simulink model "LoesungSimulink_MechanikR2020"  (R2020a)
settings: Solver=ode1  StartTime=0.0  StopTime=10.0  FixedStep=0.0001  RelTol=1e-3
undefined symbols (not defined in the file): D
settings Model: Creator=PM  LastModifiedBy=PM
settings DebuggingCC: UnconnectedInputMsg=none  UnconnectedOutputMsg=none  UnconnectedLineMsg=none
settings ModelReferenceCC: EnableRefExpFcnMdlSchedulingChecks=off
settings RTWCC: Description=Generic Real-Time Target

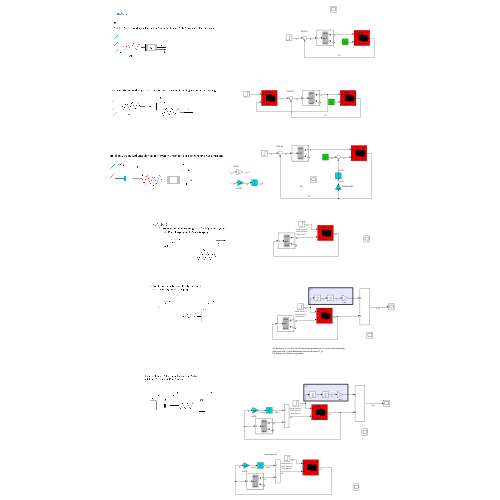
[thumbnail: Simulink's stored preview of the top-level diagram]
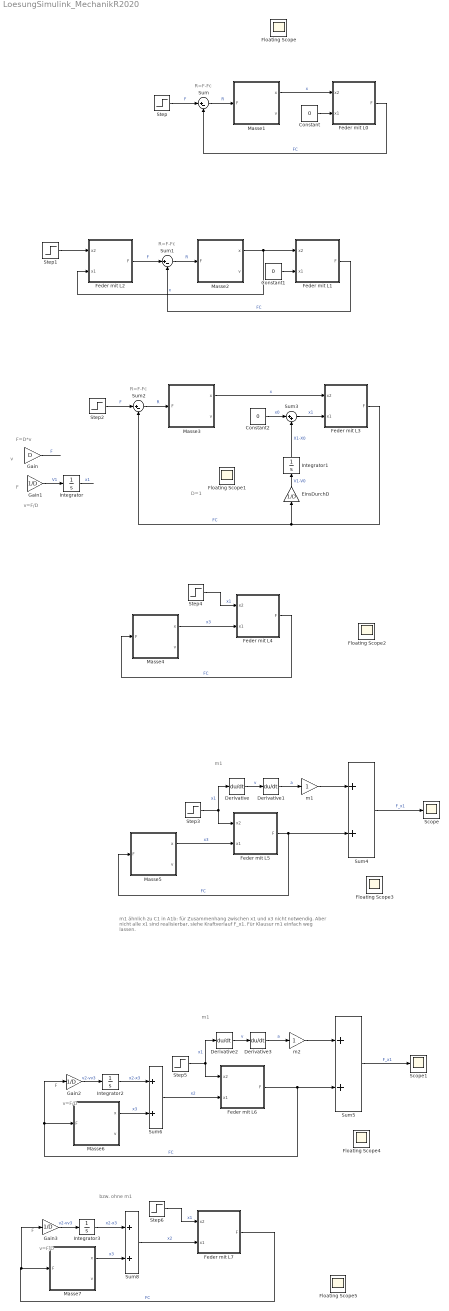
== system LoesungSimulink_MechanikR2020 ==
  note: m1
  note: m1 ähnlich zu C1 in  A1b: für Zusammenhang zwischen x1 und x3 nicht notwendig.
      | Aber nicht alle x1 sind realisierbar, siehe Kraftverlauf F_x1.
      | Für Klausur m1 einfach weg lassen.
  note: D=1
  note: F=D*v
  note: F
  note: v
  note: R=F-Fc
  note: R=F-Fc
  note: R=F-Fc
  note: v=F/D
  note: m1
  note: bzw. ohne m1
  note: F
  note: v=F/D
  note: F
  note: v=F/D
  " Feder mit L0" : Subsystem  mask{C=1, L0=0}
      mask prompts: C "Spring Constant C [N/m]"; L0 "Length of Spring if no force is applied L0 [m]"
      mask help:
      | If no force F is applied, the spring has the length L0.
      |
      | F=C*sign(x2-x1-L0)*((x2-x1-L0)
      mask Display:
      | plot(20,0)
      | plot(90,100)
      | plot([60,60],[25,30])
      | plot([60,80],[30,32])
      | plot([80,40],[32,36])
      | plot([40,80],[36,40])
      | plot([80,40],[40,44])
      | plot([40,80],[44,48])
      | plot([80,40],[48,52])
      | plot([40,80],[52,56])
      | plot([80,40],[56,60])
      | plot([40,80],[60,64])
      | plot([80,40],[64,68])
      | plot([40,60],[68,70])
      | plot([60,60],[70,75])
      | 
      | 
      | port_label ('output',1,'F')
      | port_label ('input',1,'x2')
      | port_label ('input',2,'x1')
      | 
      | text(40,10,['C=',num2str(C)])
      | text(40,90,['L0=',num2str(L0)])
  " Feder mit L1" : Subsystem  mask{C=1, L0=0}
      mask prompts: C "Spring Constant C [N/m]"; L0 "Length of Spring if no force is applied L0 [m]"
      mask help:
      | If no force F is applied, the spring has the length L0.
      |
      | F=C*sign(x2-x1-L0)*((x2-x1-L0)
      mask Display:
      | plot(20,0)
      | plot(90,100)
      | plot([60,60],[25,30])
      | plot([60,80],[30,32])
      | plot([80,40],[32,36])
      | plot([40,80],[36,40])
      | plot([80,40],[40,44])
      | plot([40,80],[44,48])
      | plot([80,40],[48,52])
      | plot([40,80],[52,56])
      | plot([80,40],[56,60])
      | plot([40,80],[60,64])
      | plot([80,40],[64,68])
      | plot([40,60],[68,70])
      | plot([60,60],[70,75])
      | 
      | 
      | port_label ('output',1,'F')
      | port_label ('input',1,'x2')
      | port_label ('input',2,'x1')
      | 
      | text(40,10,['C=',num2str(C)])
      | text(40,90,['L0=',num2str(L0)])
  " Feder mit L2" : Subsystem  mask{C=1, L0=0}
      mask prompts: C "Spring Constant C [N/m]"; L0 "Length of Spring if no force is applied L0 [m]"
      mask help:
      | If no force F is applied, the spring has the length L0.
      |
      | F=C*sign(x2-x1-L0)*((x2-x1-L0)
      mask Display:
      | plot(20,0)
      | plot(90,100)
      | plot([60,60],[25,30])
      | plot([60,80],[30,32])
      | plot([80,40],[32,36])
      | plot([40,80],[36,40])
      | plot([80,40],[40,44])
      | plot([40,80],[44,48])
      | plot([80,40],[48,52])
      | plot([40,80],[52,56])
      | plot([80,40],[56,60])
      | plot([40,80],[60,64])
      | plot([80,40],[64,68])
      | plot([40,60],[68,70])
      | plot([60,60],[70,75])
      | 
      | 
      | port_label ('output',1,'F')
      | port_label ('input',1,'x2')
      | port_label ('input',2,'x1')
      | 
      | text(40,10,['C=',num2str(C)])
      | text(40,90,['L0=',num2str(L0)])
  " Feder mit L3" : Subsystem  mask{C=1, L0=0}
      mask prompts: C "Spring Constant C [N/m]"; L0 "Length of Spring if no force is applied L0 [m]"
      mask help:
      | If no force F is applied, the spring has the length L0.
      |
      | F=C*sign(x2-x1-L0)*((x2-x1-L0)
      mask Display:
      | plot(20,0)
      | plot(90,100)
      | plot([60,60],[25,30])
      | plot([60,80],[30,32])
      | plot([80,40],[32,36])
      | plot([40,80],[36,40])
      | plot([80,40],[40,44])
      | plot([40,80],[44,48])
      | plot([80,40],[48,52])
      | plot([40,80],[52,56])
      | plot([80,40],[56,60])
      | plot([40,80],[60,64])
      | plot([80,40],[64,68])
      | plot([40,60],[68,70])
      | plot([60,60],[70,75])
      | 
      | 
      | port_label ('output',1,'F')
      | port_label ('input',1,'x2')
      | port_label ('input',2,'x1')
      | 
      | text(40,10,['C=',num2str(C)])
      | text(40,90,['L0=',num2str(L0)])
  " Feder mit L4" : Subsystem  mask{C=1, L0=1}
      mask prompts: C "Spring Constant C [N/m]"; L0 "Length of Spring if no force is applied L0 [m]"
      mask help:
      | If no force F is applied, the spring has the length L0.
      |
      | F=C*sign(x2-x1-L0)*((x2-x1-L0)
      mask Display:
      | plot(20,0)
      | plot(90,100)
      | plot([60,60],[25,30])
      | plot([60,80],[30,32])
      | plot([80,40],[32,36])
      | plot([40,80],[36,40])
      | plot([80,40],[40,44])
      | plot([40,80],[44,48])
      | plot([80,40],[48,52])
      | plot([40,80],[52,56])
      | plot([80,40],[56,60])
      | plot([40,80],[60,64])
      | plot([80,40],[64,68])
      | plot([40,60],[68,70])
      | plot([60,60],[70,75])
      | 
      | 
      | port_label ('output',1,'F')
      | port_label ('input',1,'x2')
      | port_label ('input',2,'x1')
      | 
      | text(40,10,['C=',num2str(C)])
      | text(40,90,['L0=',num2str(L0)])
  " Feder mit L5" : Subsystem  mask{C=1, L0=1}
      mask prompts: C "Spring Constant C [N/m]"; L0 "Length of Spring if no force is applied L0 [m]"
      mask help:
      | If no force F is applied, the spring has the length L0.
      |
      | F=C*sign(x2-x1-L0)*((x2-x1-L0)
      mask Display:
      | plot(20,0)
      | plot(90,100)
      | plot([60,60],[25,30])
      | plot([60,80],[30,32])
      | plot([80,40],[32,36])
      | plot([40,80],[36,40])
      | plot([80,40],[40,44])
      | plot([40,80],[44,48])
      | plot([80,40],[48,52])
      | plot([40,80],[52,56])
      | plot([80,40],[56,60])
      | plot([40,80],[60,64])
      | plot([80,40],[64,68])
      | plot([40,60],[68,70])
      | plot([60,60],[70,75])
      | 
      | 
      | port_label ('output',1,'F')
      | port_label ('input',1,'x2')
      | port_label ('input',2,'x1')
      | 
      | text(40,10,['C=',num2str(C)])
      | text(40,90,['L0=',num2str(L0)])
  " Feder mit L6" : Subsystem  mask{C=1, L0=1}
      mask prompts: C "Spring Constant C [N/m]"; L0 "Length of Spring if no force is applied L0 [m]"
      mask help:
      | If no force F is applied, the spring has the length L0.
      |
      | F=C*sign(x2-x1-L0)*((x2-x1-L0)
      mask Display:
      | plot(20,0)
      | plot(90,100)
      | plot([60,60],[25,30])
      | plot([60,80],[30,32])
      | plot([80,40],[32,36])
      | plot([40,80],[36,40])
      | plot([80,40],[40,44])
      | plot([40,80],[44,48])
      | plot([80,40],[48,52])
      | plot([40,80],[52,56])
      | plot([80,40],[56,60])
      | plot([40,80],[60,64])
      | plot([80,40],[64,68])
      | plot([40,60],[68,70])
      | plot([60,60],[70,75])
      | 
      | 
      | port_label ('output',1,'F')
      | port_label ('input',1,'x2')
      | port_label ('input',2,'x1')
      | 
      | text(40,10,['C=',num2str(C)])
      | text(40,90,['L0=',num2str(L0)])
  " Feder mit L7" : Subsystem  mask{C=1, L0=1}
      mask prompts: C "Spring Constant C [N/m]"; L0 "Length of Spring if no force is applied L0 [m]"
      mask help:
      | If no force F is applied, the spring has the length L0.
      |
      | F=C*sign(x2-x1-L0)*((x2-x1-L0)
      mask Display:
      | plot(20,0)
      | plot(90,100)
      | plot([60,60],[25,30])
      | plot([60,80],[30,32])
      | plot([80,40],[32,36])
      | plot([40,80],[36,40])
      | plot([80,40],[40,44])
      | plot([40,80],[44,48])
      | plot([80,40],[48,52])
      | plot([40,80],[52,56])
      | plot([80,40],[56,60])
      | plot([40,80],[60,64])
      | plot([80,40],[64,68])
      | plot([40,60],[68,70])
      | plot([60,60],[70,75])
      | 
      | 
      | port_label ('output',1,'F')
      | port_label ('input',1,'x2')
      | port_label ('input',2,'x1')
      | 
      | text(40,10,['C=',num2str(C)])
      | text(40,90,['L0=',num2str(L0)])
  Constant : Constant  Value=0
  Constant1 : Constant  Value=0
  Constant2 : Constant  Value=0
  Derivative{,1..3} (4 alike) : Derivative
  EinsDurchD : Gain  Gain=1/D
  Floating Scope{,1..5} (6 alike) : Scope
      settings: Floating=on
  Gain : Gain  Gain=D
  Gain1 : Gain  Gain=1/D
  Gain2 : Gain  Gain=1/D
  Gain3 : Gain  Gain=1/D
  Integrator{,1..3} (4 alike) : Integrator
  Masse1 : Subsystem  mask{m=1, v0=0, x0=0}
      mask prompts: m "Masse m"; v0 "Anfangsgeschwindigkeit v_0"; x0 "Anfangsposition x_0"
      mask help:
      | Calculates the position s and the velocity v of a mass as a function of the Force F and the initial velocity v_0 and initial position s_0.
      | Berechnet die Position und die Geschwindigkeit eines Köpers mit der Masse m. Auf den Köper wirkt die Kraft F. Die Anfangsposition ist s_0, die Anfangsgeschwindigkeit ist v_0.
      mask Display:
      | plot(0,0)
      | plot(100,100)
      | patch([35 35 70 70],[10 90 90 10],[0.7,0.7,0.7])
      | text(40,80,['x0=',num2str(x0)])
      | text(40,50,['m=',num2str(m)])
      | text(40,20,['v0=',num2str(v0)])
      | plot([70 80],[70 70])
      | patch([80 80 85],[65 75 70],[0 0 0])
      | plot([15 35],[50 50])
      | patch([30 30 35],[45 55 50],[0 0 0])
      | plot([70 80],[30 30])
      | patch([80 80 85],[25 35 30],[0 0 0])
      | port_label ('output',1,'x')
      | port_label ('output',2,'v')
      | port_label ('input',1,'F')
  Masse2 : Subsystem  mask{m=1, v0=0, x0=0}
      mask prompts: m "Masse m"; v0 "Anfangsgeschwindigkeit v_0"; x0 "Anfangsposition x_0"
      mask help:
      | Calculates the position s and the velocity v of a mass as a function of the Force F and the initial velocity v_0 and initial position s_0.
      | Berechnet die Position und die Geschwindigkeit eines Köpers mit der Masse m. Auf den Köper wirkt die Kraft F. Die Anfangsposition ist s_0, die Anfangsgeschwindigkeit ist v_0.
      mask Display:
      | plot(0,0)
      | plot(100,100)
      | patch([35 35 70 70],[10 90 90 10],[0.7,0.7,0.7])
      | text(40,80,['x0=',num2str(x0)])
      | text(40,50,['m=',num2str(m)])
      | text(40,20,['v0=',num2str(v0)])
      | plot([70 80],[70 70])
      | patch([80 80 85],[65 75 70],[0 0 0])
      | plot([15 35],[50 50])
      | patch([30 30 35],[45 55 50],[0 0 0])
      | plot([70 80],[30 30])
      | patch([80 80 85],[25 35 30],[0 0 0])
      | port_label ('output',1,'x')
      | port_label ('output',2,'v')
      | port_label ('input',1,'F')
  Masse3 : Subsystem  mask{m=1, v0=0, x0=0}
      mask prompts: m "Masse m"; v0 "Anfangsgeschwindigkeit v_0"; x0 "Anfangsposition x_0"
      mask help:
      | Calculates the position s and the velocity v of a mass as a function of the Force F and the initial velocity v_0 and initial position s_0.
      | Berechnet die Position und die Geschwindigkeit eines Köpers mit der Masse m. Auf den Köper wirkt die Kraft F. Die Anfangsposition ist s_0, die Anfangsgeschwindigkeit ist v_0.
      mask Display:
      | plot(0,0)
      | plot(100,100)
      | patch([35 35 70 70],[10 90 90 10],[0.7,0.7,0.7])
      | text(40,80,['x0=',num2str(x0)])
      | text(40,50,['m=',num2str(m)])
      | text(40,20,['v0=',num2str(v0)])
      | plot([70 80],[70 70])
      | patch([80 80 85],[65 75 70],[0 0 0])
      | plot([15 35],[50 50])
      | patch([30 30 35],[45 55 50],[0 0 0])
      | plot([70 80],[30 30])
      | patch([80 80 85],[25 35 30],[0 0 0])
      | port_label ('output',1,'x')
      | port_label ('output',2,'v')
      | port_label ('input',1,'F')
  Masse4 : Subsystem  mask{m=1, v0=0, x0=0}
      mask prompts: m "Masse m"; v0 "Anfangsgeschwindigkeit v_0"; x0 "Anfangsposition x_0"
      mask help:
      | Calculates the position s and the velocity v of a mass as a function of the Force F and the initial velocity v_0 and initial position s_0.
      | Berechnet die Position und die Geschwindigkeit eines Köpers mit der Masse m. Auf den Köper wirkt die Kraft F. Die Anfangsposition ist s_0, die Anfangsgeschwindigkeit ist v_0.
      mask Display:
      | plot(0,0)
      | plot(100,100)
      | patch([35 35 70 70],[10 90 90 10],[0.7,0.7,0.7])
      | text(40,80,['x0=',num2str(x0)])
      | text(40,50,['m=',num2str(m)])
      | text(40,20,['v0=',num2str(v0)])
      | plot([70 80],[70 70])
      | patch([80 80 85],[65 75 70],[0 0 0])
      | plot([15 35],[50 50])
      | patch([30 30 35],[45 55 50],[0 0 0])
      | plot([70 80],[30 30])
      | patch([80 80 85],[25 35 30],[0 0 0])
      | port_label ('output',1,'x')
      | port_label ('output',2,'v')
      | port_label ('input',1,'F')
  Masse5 : Subsystem  mask{m=1, v0=0, x0=0}
      mask prompts: m "Masse m"; v0 "Anfangsgeschwindigkeit v_0"; x0 "Anfangsposition x_0"
      mask help:
      | Calculates the position s and the velocity v of a mass as a function of the Force F and the initial velocity v_0 and initial position s_0.
      | Berechnet die Position und die Geschwindigkeit eines Köpers mit der Masse m. Auf den Köper wirkt die Kraft F. Die Anfangsposition ist s_0, die Anfangsgeschwindigkeit ist v_0.
      mask Display:
      | plot(0,0)
      | plot(100,100)
      | patch([35 35 70 70],[10 90 90 10],[0.7,0.7,0.7])
      | text(40,80,['x0=',num2str(x0)])
      | text(40,50,['m=',num2str(m)])
      | text(40,20,['v0=',num2str(v0)])
      | plot([70 80],[70 70])
      | patch([80 80 85],[65 75 70],[0 0 0])
      | plot([15 35],[50 50])
      | patch([30 30 35],[45 55 50],[0 0 0])
      | plot([70 80],[30 30])
      | patch([80 80 85],[25 35 30],[0 0 0])
      | port_label ('output',1,'x')
      | port_label ('output',2,'v')
      | port_label ('input',1,'F')
  Masse6 : Subsystem  mask{m=1, v0=0, x0=0}
      mask prompts: m "Masse m"; v0 "Anfangsgeschwindigkeit v_0"; x0 "Anfangsposition x_0"
      mask help:
      | Calculates the position s and the velocity v of a mass as a function of the Force F and the initial velocity v_0 and initial position s_0.
      | Berechnet die Position und die Geschwindigkeit eines Köpers mit der Masse m. Auf den Köper wirkt die Kraft F. Die Anfangsposition ist s_0, die Anfangsgeschwindigkeit ist v_0.
      mask Display:
      | plot(0,0)
      | plot(100,100)
      | patch([35 35 70 70],[10 90 90 10],[0.7,0.7,0.7])
      | text(40,80,['x0=',num2str(x0)])
      | text(40,50,['m=',num2str(m)])
      | text(40,20,['v0=',num2str(v0)])
      | plot([70 80],[70 70])
      | patch([80 80 85],[65 75 70],[0 0 0])
      | plot([15 35],[50 50])
      | patch([30 30 35],[45 55 50],[0 0 0])
      | plot([70 80],[30 30])
      | patch([80 80 85],[25 35 30],[0 0 0])
      | port_label ('output',1,'x')
      | port_label ('output',2,'v')
      | port_label ('input',1,'F')
  Masse7 : Subsystem  mask{m=1, v0=0, x0=0}
      mask prompts: m "Masse m"; v0 "Anfangsgeschwindigkeit v_0"; x0 "Anfangsposition x_0"
      mask help:
      | Calculates the position s and the velocity v of a mass as a function of the Force F and the initial velocity v_0 and initial position s_0.
      | Berechnet die Position und die Geschwindigkeit eines Köpers mit der Masse m. Auf den Köper wirkt die Kraft F. Die Anfangsposition ist s_0, die Anfangsgeschwindigkeit ist v_0.
      mask Display:
      | plot(0,0)
      | plot(100,100)
      | patch([35 35 70 70],[10 90 90 10],[0.7,0.7,0.7])
      | text(40,80,['x0=',num2str(x0)])
      | text(40,50,['m=',num2str(m)])
      | text(40,20,['v0=',num2str(v0)])
      | plot([70 80],[70 70])
      | patch([80 80 85],[65 75 70],[0 0 0])
      | plot([15 35],[50 50])
      | patch([30 30 35],[45 55 50],[0 0 0])
      | plot([70 80],[30 30])
      | patch([80 80 85],[25 35 30],[0 0 0])
      | port_label ('output',1,'x')
      | port_label ('output',2,'v')
      | port_label ('input',1,'F')
  Scope : Scope
  Scope1 : Scope
  Step : Step  SampleTime=0
  Step1 : Step  SampleTime=0
  Step2 : Step  SampleTime=0
  Step{3..6} (4 alike) : Step  Before=1  After=2  SampleTime=0
      settings: AttributesFormatString=initial value=%<Before>\nfinal value=%<After>\nstep time=%<Time>
  Sum : Sum  Inputs=|+-
  Sum1 : Sum  Inputs=|+-
  Sum2 : Sum  Inputs=|+-
  Sum3 : Sum  Inputs=|++
  Sum{4..6,8} (4 alike) : Sum
  m1 : Gain
  m2 : Gain
  wires:
  Constant/1 -> " Feder mit L0"/2(x1)
  Masse1/1(x) -> " Feder mit L0"/1(x2)  "x"
  Sum/1 -> Masse1/1(F)  "R"
  Step/1 -> Sum/1  "F"
  " Feder mit L0"/1(F) -> Sum/2  "FC"
  Constant1/1 -> " Feder mit L1"/2(x1)
  " Feder mit L1"/1(F) -> Sum1/2  "FC"
  Sum1/1 -> Masse2/1(F)  "R"
  Masse2/1(x) -> " Feder mit L2"/2(x1), " Feder mit L1"/1(x2)  "x"
  " Feder mit L2"/1(F) -> Sum1/1  "F"
  Step1/1 -> " Feder mit L2"/1(x2)
  " Feder mit L3"/1(F) -> EinsDurchD/1, Sum2/2  "FC"
  Sum2/1 -> Masse3/1(F)  "R"
  Masse3/1(x) -> " Feder mit L3"/1(x2)  "x"
  Step2/1 -> Sum2/1  "F"
  ? -> Gain/1
  Gain/1 -> ?  "F"
  ? -> Gain1/1
  Gain1/1 -> Integrator/1  "V1"
  Integrator/1 -> ?  "x1"
  EinsDurchD/1 -> Integrator1/1  "V1-V0"
  Sum3/1 -> " Feder mit L3"/2(x1)  "x1"
  Integrator1/1 -> Sum3/2  "X1-X0"
  Constant2/1 -> Sum3/1  "x0"
  Masse4/1(x) -> " Feder mit L4"/2(x1)  "x3"
  Step4/1 -> " Feder mit L4"/1(x2)  "x1"
  " Feder mit L4"/1(F) -> Masse4/1(F)  "FC"
  Step3/1 -> " Feder mit L5"/1(x2), Derivative/1  "x1"
  Masse5/1(x) -> " Feder mit L5"/2(x1)  "x3"
  " Feder mit L5"/1(F) -> Sum4/2, Masse5/1(F)  "FC"
  Derivative/1 -> Derivative1/1  "v"
  Derivative1/1 -> m1/1  "a"
  m1/1 -> Sum4/1
  Sum4/1 -> Scope/1  "F_x1"
  Sum5/1 -> Scope1/1  "F_x1"
  m2/1 -> Sum5/1
  Derivative3/1 -> m2/1  "a"
  " Feder mit L6"/1(F) -> Gain2/1, Masse6/1(F), Sum5/2  "FC"
  Sum6/1 -> " Feder mit L6"/2(x1)  "x2"
  Step5/1 -> " Feder mit L6"/1(x2), Derivative2/1  "x1"
  Derivative2/1 -> Derivative3/1  "v"
  Integrator2/1 -> Sum6/1  "x2-x3"
  Gain2/1 -> Integrator2/1  "v2-vv3"
  Masse6/1(x) -> Sum6/2  "x3"
  Integrator3/1 -> Sum8/1  "x2-x3"
  Gain3/1 -> Integrator3/1  "v2-vv3"
  " Feder mit L7"/1(F) -> Gain3/1, Masse7/1(F)  "FC"
  Masse7/1(x) -> Sum8/2  "x3"
  Step6/1 -> " Feder mit L7"/1(x2)  "x1"
  Sum8/1 -> " Feder mit L7"/2(x1)  "x2"

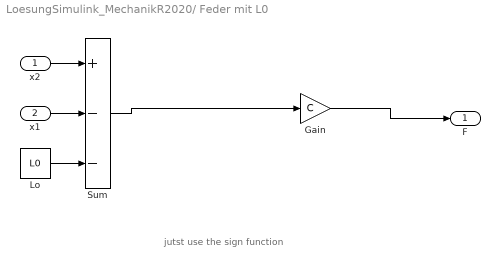
== system LoesungSimulink_MechanikR2020/ Feder mit L0 ==
  note: jutst use the sign function
  x2 : Inport
  x1 : Inport  Port=2
  Gain : Gain  Gain=C
  Lo : Constant  Value=L0
  Sum : Sum  Inputs=+--
  F : Outport  VectorParamsAs1DForOutWhenUnconnected=off
  wires:
  Gain/1 -> F/1
  Sum/1 -> Gain/1
  Lo/1 -> Sum/3
  x1/1 -> Sum/2
  x2/1 -> Sum/1

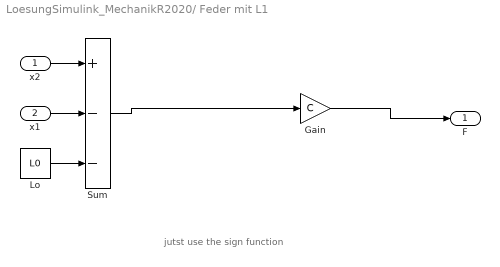
== system LoesungSimulink_MechanikR2020/ Feder mit L1 ==
  note: jutst use the sign function
  x2 : Inport
  x1 : Inport  Port=2
  Gain : Gain  Gain=C
  Lo : Constant  Value=L0
  Sum : Sum  Inputs=+--
  F : Outport  VectorParamsAs1DForOutWhenUnconnected=off
  wires:
  Gain/1 -> F/1
  Sum/1 -> Gain/1
  Lo/1 -> Sum/3
  x1/1 -> Sum/2
  x2/1 -> Sum/1

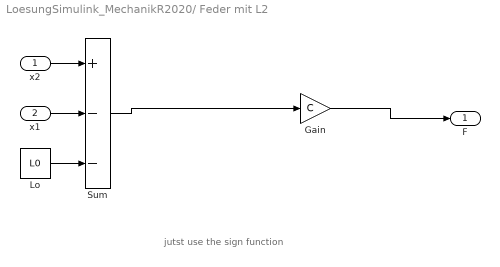
== system LoesungSimulink_MechanikR2020/ Feder mit L2 ==
  note: jutst use the sign function
  x2 : Inport
  x1 : Inport  Port=2
  Gain : Gain  Gain=C
  Lo : Constant  Value=L0
  Sum : Sum  Inputs=+--
  F : Outport  VectorParamsAs1DForOutWhenUnconnected=off
  wires:
  Gain/1 -> F/1
  Sum/1 -> Gain/1
  Lo/1 -> Sum/3
  x1/1 -> Sum/2
  x2/1 -> Sum/1

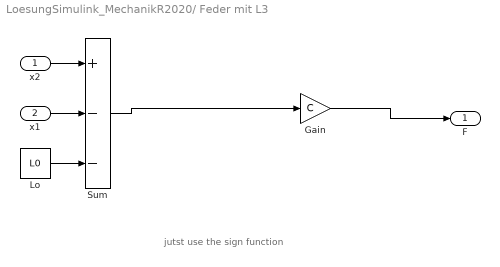
== system LoesungSimulink_MechanikR2020/ Feder mit L3 ==
  note: jutst use the sign function
  x2 : Inport
  x1 : Inport  Port=2
  Gain : Gain  Gain=C
  Lo : Constant  Value=L0
  Sum : Sum  Inputs=+--
  F : Outport  VectorParamsAs1DForOutWhenUnconnected=off
  wires:
  Gain/1 -> F/1
  Sum/1 -> Gain/1
  Lo/1 -> Sum/3
  x1/1 -> Sum/2
  x2/1 -> Sum/1

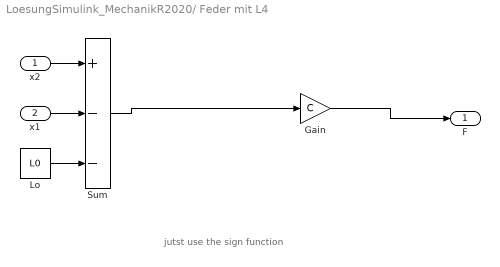
== system LoesungSimulink_MechanikR2020/ Feder mit L4 ==
  note: jutst use the sign function
  x2 : Inport
  x1 : Inport  Port=2
  Gain : Gain  Gain=C
  Lo : Constant  Value=L0
  Sum : Sum  Inputs=+--
  F : Outport  VectorParamsAs1DForOutWhenUnconnected=off
  wires:
  Gain/1 -> F/1
  Sum/1 -> Gain/1
  Lo/1 -> Sum/3
  x1/1 -> Sum/2
  x2/1 -> Sum/1

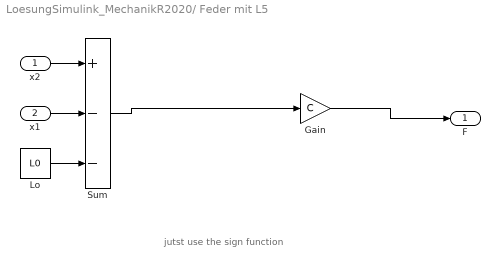
== system LoesungSimulink_MechanikR2020/ Feder mit L5 ==
  note: jutst use the sign function
  x2 : Inport
  x1 : Inport  Port=2
  Gain : Gain  Gain=C
  Lo : Constant  Value=L0
  Sum : Sum  Inputs=+--
  F : Outport  VectorParamsAs1DForOutWhenUnconnected=off
  wires:
  Gain/1 -> F/1
  Sum/1 -> Gain/1
  Lo/1 -> Sum/3
  x1/1 -> Sum/2
  x2/1 -> Sum/1

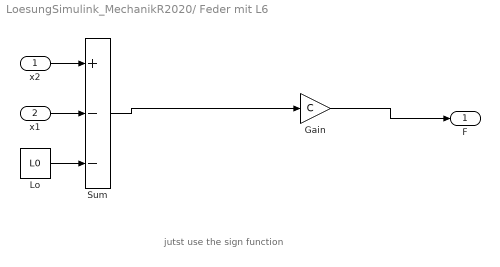
== system LoesungSimulink_MechanikR2020/ Feder mit L6 ==
  note: jutst use the sign function
  x2 : Inport
  x1 : Inport  Port=2
  Gain : Gain  Gain=C
  Lo : Constant  Value=L0
  Sum : Sum  Inputs=+--
  F : Outport  VectorParamsAs1DForOutWhenUnconnected=off
  wires:
  Gain/1 -> F/1
  Sum/1 -> Gain/1
  Lo/1 -> Sum/3
  x1/1 -> Sum/2
  x2/1 -> Sum/1

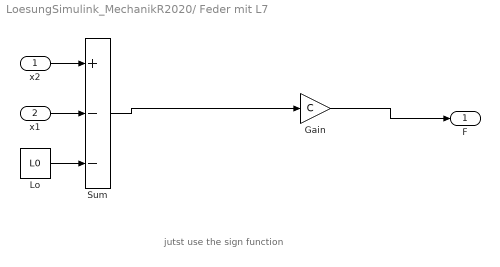
== system LoesungSimulink_MechanikR2020/ Feder mit L7 ==
  note: jutst use the sign function
  x2 : Inport
  x1 : Inport  Port=2
  Gain : Gain  Gain=C
  Lo : Constant  Value=L0
  Sum : Sum  Inputs=+--
  F : Outport  VectorParamsAs1DForOutWhenUnconnected=off
  wires:
  Gain/1 -> F/1
  Sum/1 -> Gain/1
  Lo/1 -> Sum/3
  x1/1 -> Sum/2
  x2/1 -> Sum/1

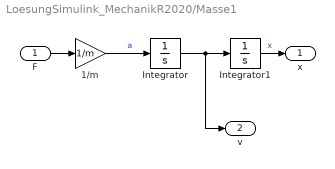
== system LoesungSimulink_MechanikR2020/Masse1 ==
  F : Inport
  1/m : Gain  Gain=1/m
  Integrator : Integrator  InitialCondition=v0
  Integrator1 : Integrator  InitialCondition=x0
  x : Outport  VectorParamsAs1DForOutWhenUnconnected=off
  v : Outport  Port=2  VectorParamsAs1DForOutWhenUnconnected=off
  wires:
  Integrator1/1 -> x/1  "x"
  F/1 -> 1/m/1
  Integrator/1 -> v/1, Integrator1/1
  1/m/1 -> Integrator/1  "a"

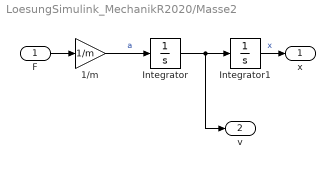
== system LoesungSimulink_MechanikR2020/Masse2 ==
  F : Inport
  1/m : Gain  Gain=1/m
  Integrator : Integrator  InitialCondition=v0
  Integrator1 : Integrator  InitialCondition=x0
  x : Outport  VectorParamsAs1DForOutWhenUnconnected=off
  v : Outport  Port=2  VectorParamsAs1DForOutWhenUnconnected=off
  wires:
  Integrator1/1 -> x/1  "x"
  F/1 -> 1/m/1
  Integrator/1 -> v/1, Integrator1/1
  1/m/1 -> Integrator/1  "a"

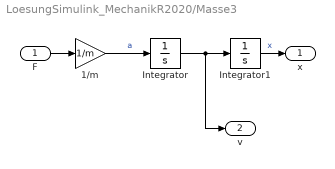
== system LoesungSimulink_MechanikR2020/Masse3 ==
  F : Inport
  1/m : Gain  Gain=1/m
  Integrator : Integrator  InitialCondition=v0
  Integrator1 : Integrator  InitialCondition=x0
  x : Outport  VectorParamsAs1DForOutWhenUnconnected=off
  v : Outport  Port=2  VectorParamsAs1DForOutWhenUnconnected=off
  wires:
  Integrator1/1 -> x/1  "x"
  F/1 -> 1/m/1
  Integrator/1 -> v/1, Integrator1/1
  1/m/1 -> Integrator/1  "a"

== system LoesungSimulink_MechanikR2020/Masse4 ==
  F : Inport
  1/m : Gain  Gain=1/m
  Integrator : Integrator  InitialCondition=v0
  Integrator1 : Integrator  InitialCondition=x0
  x : Outport  VectorParamsAs1DForOutWhenUnconnected=off
  v : Outport  Port=2  VectorParamsAs1DForOutWhenUnconnected=off
  wires:
  Integrator1/1 -> x/1  "x"
  F/1 -> 1/m/1
  Integrator/1 -> v/1, Integrator1/1
  1/m/1 -> Integrator/1  "a"

== system LoesungSimulink_MechanikR2020/Masse5 ==
  F : Inport
  1/m : Gain  Gain=1/m
  Integrator : Integrator  InitialCondition=v0
  Integrator1 : Integrator  InitialCondition=x0
  x : Outport  VectorParamsAs1DForOutWhenUnconnected=off
  v : Outport  Port=2  VectorParamsAs1DForOutWhenUnconnected=off
  wires:
  Integrator1/1 -> x/1  "x"
  F/1 -> 1/m/1
  Integrator/1 -> v/1, Integrator1/1
  1/m/1 -> Integrator/1  "a"

== system LoesungSimulink_MechanikR2020/Masse6 ==
  F : Inport
  1/m : Gain  Gain=1/m
  Integrator : Integrator  InitialCondition=v0
  Integrator1 : Integrator  InitialCondition=x0
  x : Outport  VectorParamsAs1DForOutWhenUnconnected=off
  v : Outport  Port=2  VectorParamsAs1DForOutWhenUnconnected=off
  wires:
  Integrator1/1 -> x/1  "x"
  F/1 -> 1/m/1
  Integrator/1 -> v/1, Integrator1/1
  1/m/1 -> Integrator/1  "a"

== system LoesungSimulink_MechanikR2020/Masse7 ==
  F : Inport
  1/m : Gain  Gain=1/m
  Integrator : Integrator  InitialCondition=v0
  Integrator1 : Integrator  InitialCondition=x0
  x : Outport  VectorParamsAs1DForOutWhenUnconnected=off
  v : Outport  Port=2  VectorParamsAs1DForOutWhenUnconnected=off
  wires:
  Integrator1/1 -> x/1  "x"
  F/1 -> 1/m/1
  Integrator/1 -> v/1, Integrator1/1
  1/m/1 -> Integrator/1  "a"
